simulink model "variableStop_fsm"  (R2022a)
settings: Solver=FixedStepDiscrete  StartTime=0.0  StopTime=10.0  FixedStep=0.1  RelTol=1e-3  EnableMultiTasking=on
settings Model: Creator=steve  LastModifiedBy=Nate
settings SolverCC: AlgebraicLoopSolver=TrustRegion  AutoInsertRateTranBlk=on
settings DataIOCC: LimitDataPoints=on
settings OptimizationCC: LifeSpan=inf
settings DebuggingCC: UnconnectedInputMsg=warning  UnconnectedOutputMsg=warning  UnconnectedLineMsg=warning  AllowSymbolicDim=off  SFUnexpectedBacktrackingDiag=warning  SFNoUnconditionalDefaultTransitionDiag=warning  SFExecutionAtInitializationDiag=none  ArithmeticOperatorsInVariantConditions=warning
settings SFSimCC: SimUseLocalCustomCode=off  CustomCodeUndefinedFunction=UseInterfaceOnly
settings RTWCC: RTWUseLocalCustomCode=off  DLArmComputeVersion=19.05
settings CodeAppCC: StateflowObjectComments=on
settings GRTTargetCC: TargetLangStandard=C89/C90 (ANSI)
settings ConfigComp: CovMetricSettings=dw  CovSaveCumulativeToWorkspaceVar=on  CovSaveSingleToWorkspaceVar=on  CovExternalEMLEnable=off  CovSFcnEnable=off

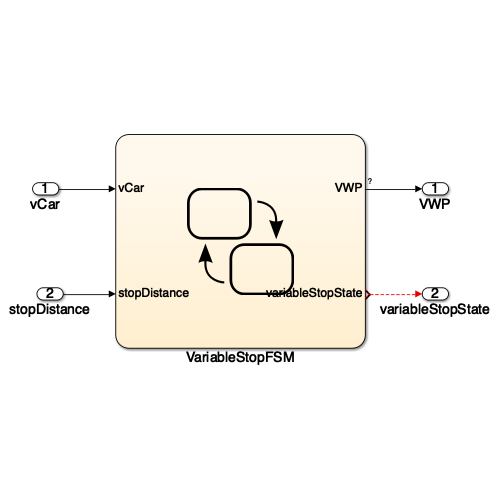
[thumbnail: Simulink's stored preview of the top-level diagram]
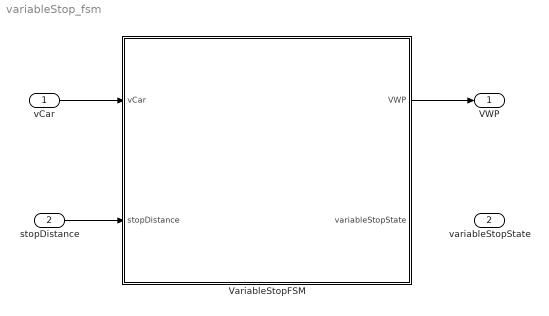
== system variableStop_fsm ==
  vCar : Inport
  stopDistance : Inport  Port=2
  VariableStopFSM : Stateflow chart  TreatAsAtomicUnit=on
  VWP : Outport
  variableStopState : Outport  Port=2
  wires:
  ? -> variableStopState/1
  VariableStopFSM/1(VWP) -> VWP/1
  vCar/1 -> VariableStopFSM/1(vCar)
  stopDistance/1 -> VariableStopFSM/2(stopDistance)

== stateflow chart variableStop_fsm/VariableStopFSM ==
  state wait_for_variableStop_enable
    en:  variableStopState = 0;
  state wait_for_zero_velocity1
    en:  variableStopState = 1;
  state wait_while_curObstacle_is_present
    en:  variableStopState = 2;
    en: curObstacle = sort(ActiveObjectList)
  (default) -> wait_for_variableStop_enable
  wait_for_variableStop_enable -> wait_for_variableStop_enable [order 1]
  wait_while_curObstacle_is_present -> wait_for_variableStop_enable [order 1] : [SpeedChangeEnable == false || ...
      |   ~ismember(curObstacle, ActiveObstacleList)]
      | {SubMachineRunning = false;
      | VariableStopEnable = false;}
  wait_for_zero_velocity1 -> wait_for_variableStop_enable [order 1] : [VariableStopEnable == false]
  wait_for_variableStop_enable -> wait_for_zero_velocity1 [order 2] : [VariableStopEnable == true]
      | {VWP = updateVWP(VWP, stopDistance)}
  wait_for_zero_velocity1 -> wait_for_zero_velocity1 [order 3]
  wait_for_zero_velocity1 -> wait_while_curObstacle_is_present [order 2] : [vCar == 0]
  wait_while_curObstacle_is_present -> wait_while_curObstacle_is_present [order 2]
  data: VWP output; ActiveObjectList data_store_memory; SpeedChangeEnable data_store_memory; VariableStopEnable data_store_memory; SubMachineRunning data_store_memory; curObstacle local; variableStopState output; vCar input; stopDistance input
